simulink library "motor_control_lib"  (R2025b)
settings: Solver=VariableStepAuto  StartTime=0.0  StopTime=10.0  RelTol=1e-3
settings Model: Creator=ali89  LastModifiedBy=ali89

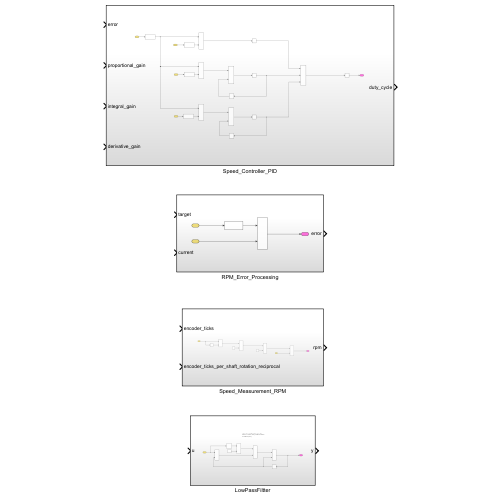
[thumbnail: Simulink's stored preview of the top-level diagram]
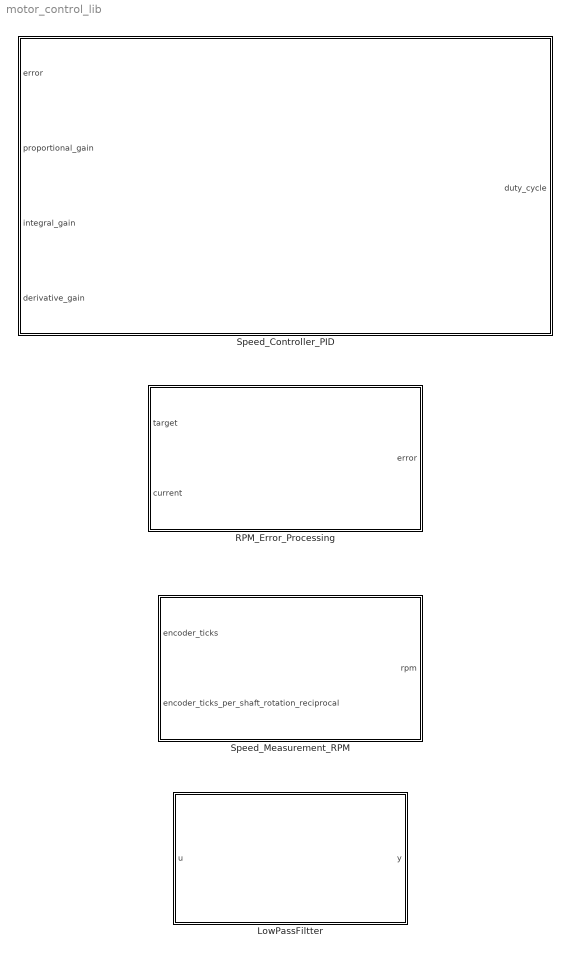
== system motor_control_lib ==
  LowPassFiltter : Subsystem
  RPM_Error_Processing : Subsystem
  Speed_Controller_PID : Subsystem
  Speed_Measurement_RPM : Subsystem

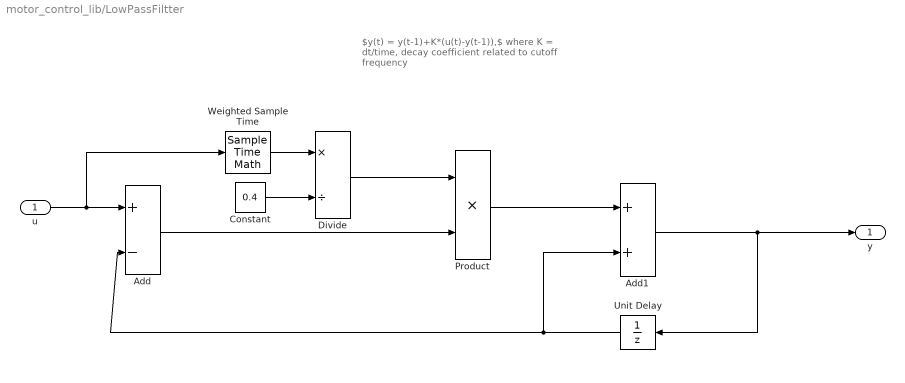
== system motor_control_lib/LowPassFiltter ==
  note: $y(t) = y(t-1)+K*(u(t)-y(t-1)),$
      | where K = dt/time, decay coefficient related to cutoff frequency
  u : Inport
  Add : Sum  Inputs=+-
  Add1 : Sum
  Constant : Constant  Value=0.4
  Divide : Product  Inputs=*/
  Product : Product
  Unit Delay : UnitDelay  SampleTime=-1  HasFrameUpgradeWarning=on
  Weighted Sample Time : SampleTimeMath  TsampMathOp=Ts Only
  y : Outport
  wires:
  Unit Delay/1 -> Add/2, Add1/2
  Add1/1 -> y/1, Unit Delay/1
  Product/1 -> Add1/1
  Add/1 -> Product/2
  Divide/1 -> Product/1
  u/1 -> Add/1, Weighted Sample Time/1
  Weighted Sample Time/1 -> Divide/1
  Constant/1 -> Divide/2

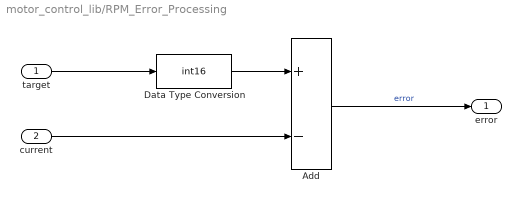
== system motor_control_lib/RPM_Error_Processing ==
  target : Inport
  current : Inport  Port=2
  Add : Sum  Inputs=+-
  Data Type Conversion : DataTypeConversion  OutDataTypeStr=int16  SaturateOnIntegerOverflow=off  RndMeth=Floor
  error : Outport
  wires:
  current/1 -> Add/2
  target/1 -> Data Type Conversion/1
  Add/1 -> error/1  "error"
  Data Type Conversion/1 -> Add/1

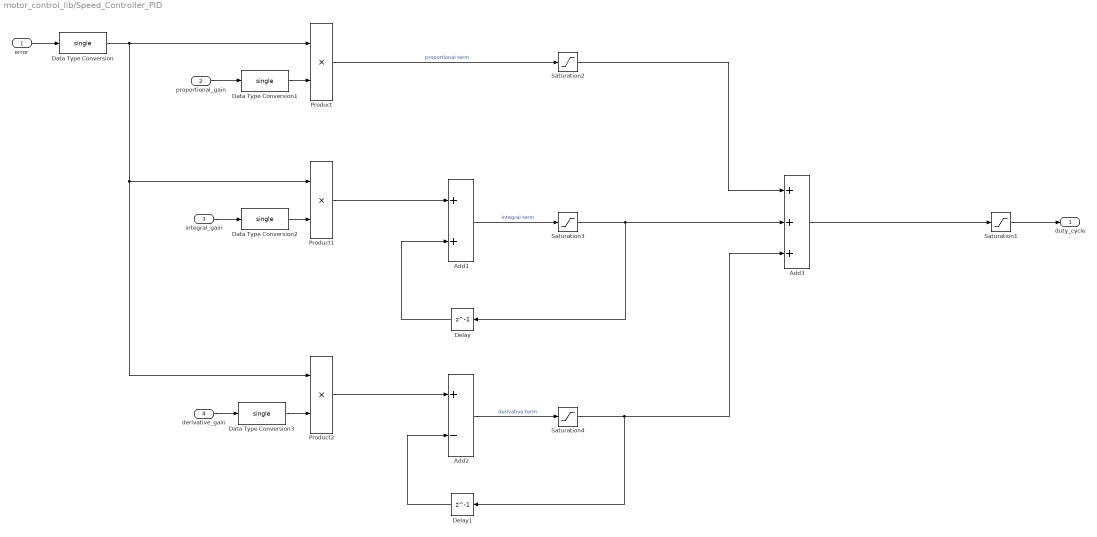
== system motor_control_lib/Speed_Controller_PID ==
  error : Inport
  proportional_gain : Inport  Port=2
  integral_gain : Inport  Port=3
  derivative_gain : Inport  Port=4
  Add1 : Sum
  Add2 : Sum  Inputs=+-
  Add3 : Sum  Inputs=+++
  Data Type Conversion{,1..3} (4 alike) : DataTypeConversion  OutDataTypeStr=single  SaturateOnIntegerOverflow=off  RndMeth=Floor
  Delay : Delay  DelayLength=1  InputProcessing=Columns as channels (frame based)
  Delay1 : Delay  DelayLength=1  InputProcessing=Columns as channels (frame based)
  Product : Product
  Product1 : Product
  Product2 : Product
  Saturation1 : Saturate  UpperLimit=255  LowerLimit=0
  Saturation2 : Saturate  UpperLimit=255  LowerLimit=-255
  Saturation3 : Saturate  UpperLimit=255  LowerLimit=-255
  Saturation4 : Saturate  UpperLimit=255  LowerLimit=-255
  duty_cycle : Outport
  wires:
  Data Type Conversion3/1 -> Product2/2
  Data Type Conversion2/1 -> Product1/2
  Data Type Conversion1/1 -> Product/2
  Data Type Conversion/1 -> Product/1, Product1/1, Product2/1
  Saturation4/1 -> Add3/3, Delay1/1
  Add2/1 -> Saturation4/1  "derivative term"
  derivative_gain/1 -> Data Type Conversion3/1
  Add1/1 -> Saturation3/1  "integral term"
  Delay/1 -> Add1/2
  Product2/1 -> Add2/1
  error/1 -> Data Type Conversion/1
  integral_gain/1 -> Data Type Conversion2/1
  Saturation3/1 -> Add3/2, Delay/1
  Product1/1 -> Add1/1
  proportional_gain/1 -> Data Type Conversion1/1
  Saturation1/1 -> duty_cycle/1
  Delay1/1 -> Add2/2
  Saturation2/1 -> Add3/1
  Product/1 -> Saturation2/1  "proportional term"
  Add3/1 -> Saturation1/1

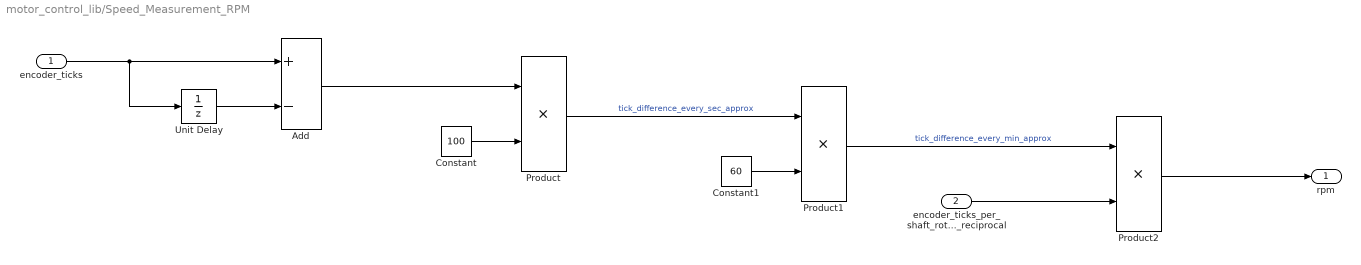
== system motor_control_lib/Speed_Measurement_RPM ==
  encoder_ticks : Inport
  encoder_ticks_per_shaft_rotation_reciprocal : Inport  Port=2
  Add : Sum  Inputs=+-
  Constant : Constant  Value=100
  Constant1 : Constant  Value=60
  Product : Product
  Product1 : Product
  Product2 : Product
  Unit Delay : UnitDelay  SampleTime=-1  HasFrameUpgradeWarning=on
  rpm : Outport
  wires:
  encoder_ticks/1 -> Unit Delay/1, Add/1
  Unit Delay/1 -> Add/2
  encoder_ticks_per_shaft_rotation_reciprocal/1 -> Product2/2
  Add/1 -> Product/1
  Constant/1 -> Product/2
  Product/1 -> Product1/1  "tick_difference_every_sec_approx"
  Constant1/1 -> Product1/2
  Product1/1 -> Product2/1  "tick_difference_every_min_approx"
  Product2/1 -> rpm/1
